simulink library "lib_Clutch_2017a"  (R2017a)
settings: Solver=VariableStepAuto  StartTime=0.0  StopTime=10.0  RelTol=1e-3
settings Model: Creator=leste  LastModifiedBy=Di Russo

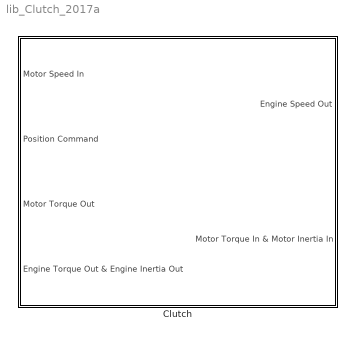
== system lib_Clutch_2017a ==
  Clutch : Subsystem
      mask Display:
      | color('red');
      | port_label('Input',1,'Motor Speed In')
      | port_label('Input',2,'Position Command')
      | port_label('Input',3,'Motor Torque Out')
      | port_label('Input',4,'Engine Trq & Inertia Out')
      | port_label('Output',1,'Engine Speed Out')
      | port_label('Output',2,'Motor Trq Inertia In')

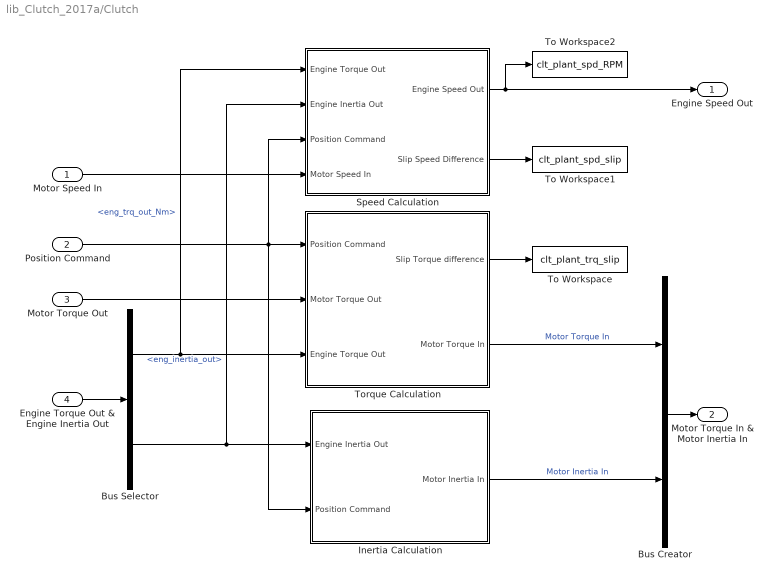
== system lib_Clutch_2017a/Clutch ==
  Motor Speed In : Inport
  Position Command : Inport  Port=2
  Motor Torque Out : Inport  Port=3
  Engine Torque Out & Engine Inertia Out : Inport  Port=4
  Bus Creator : BusCreator  Inputs=2
  Bus Selector : BusSelector  OutputSignals=eng_trq_out_Nm,eng_inertia_out
  Inertia Calculation : Subsystem
  Speed Calculation : Subsystem
  To Workspace : ToWorkspace  VariableName=clt_plant_trq_slip  SaveFormat=Timeseries  SampleTime=-1
  To Workspace1 : ToWorkspace  VariableName=clt_plant_spd_slip  SaveFormat=Timeseries  SampleTime=-1
  To Workspace2 : ToWorkspace  VariableName=clt_plant_spd_RPM  SaveFormat=Timeseries  SampleTime=-1
  Torque Calculation : Subsystem
  Engine Speed Out : Outport
  Motor Torque In & Motor Inertia In : Outport  Port=2
  wires:
  Motor Speed In/1 -> Speed Calculation/4(Motor Speed In)
  Motor Torque Out/1 -> Torque Calculation/2(Motor Torque Out)
  Speed Calculation/2(Slip Speed Difference) -> To Workspace1/1
  Bus Creator/1 -> Motor Torque In & Motor Inertia In/1
  Torque Calculation/1(Slip Torque difference) -> To Workspace/1
  Engine Torque Out & Engine Inertia Out/1 -> Bus Selector/1
  Inertia Calculation/1(Motor Inertia In) -> Bus Creator/2  "Motor Inertia In"
  Torque Calculation/2(Motor Torque In) -> Bus Creator/1  "Motor Torque In"
  Speed Calculation/1(Engine Speed Out) -> Engine Speed Out/1, To Workspace2/1
  Bus Selector/1 -> Torque Calculation/3(Engine Torque Out), Speed Calculation/1(Engine Torque Out)  "<eng_trq_out_Nm>"
  Position Command/1 -> Inertia Calculation/2(Position Command), Speed Calculation/3(Position Command), Torque Calculation/1(Position Command)
  Bus Selector/2 -> Speed Calculation/2(Engine Inertia Out), Inertia Calculation/1(Engine Inertia Out)  "<eng_inertia_out>"

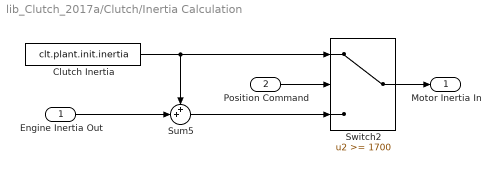
== system lib_Clutch_2017a/Clutch/Inertia Calculation ==
  Engine Inertia Out : Inport
  Position Command : Inport  Port=2
  Clutch Inertia : Constant  Value=clt.plant.init.inertia
  Sum5 : Sum  Inputs=++|  SaturateOnIntegerOverflow=on  InputSameDT=on  OutDataTypeStr=Inherit: Same as first input
  Switch2 : Switch  Threshold=1700  SaturateOnIntegerOverflow=on  InputSameDT=on
  Motor Inertia In : Outport
  wires:
  Clutch Inertia/1 -> Switch2/1, Sum5/1
  Engine Inertia Out/1 -> Sum5/2
  Position Command/1 -> Switch2/2
  Sum5/1 -> Switch2/3
  Switch2/1 -> Motor Inertia In/1

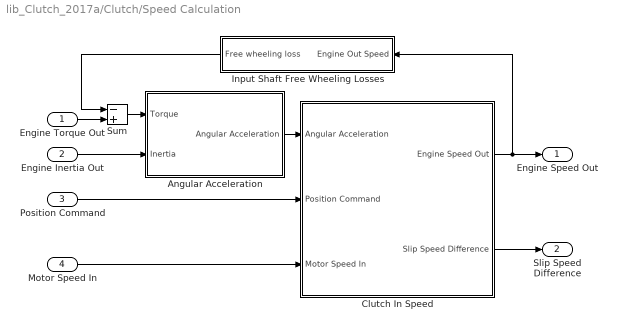
== system lib_Clutch_2017a/Clutch/Speed Calculation ==
  Engine Torque Out : Inport
  Engine Inertia Out : Inport  Port=2
  Position Command : Inport  Port=3
  Motor Speed In : Inport  Port=4
  Angular Acceleration : Subsystem
  "Clutch In Speed " : Subsystem
  Input Shaft Free Wheeling Losses : Subsystem
  Sum : Sum  Inputs=-+
  Engine Speed Out : Outport
  Slip Speed Difference : Outport  Port=2
  wires:
  "Clutch In Speed "/2(Slip Speed Difference) -> Slip Speed Difference/1
  Angular Acceleration/1(Angular Acceleration) -> "Clutch In Speed "/1(Angular Acceleration)
  Position Command/1 -> "Clutch In Speed "/2(Position Command)
  Motor Speed In/1 -> "Clutch In Speed "/3(Motor Speed In)
  Engine Inertia Out/1 -> Angular Acceleration/2(Inertia)
  Engine Torque Out/1 -> Sum/2
  "Clutch In Speed "/1(Engine Speed Out) -> Engine Speed Out/1, Input Shaft Free Wheeling Losses/1(Engine Out Speed)
  Input Shaft Free Wheeling Losses/1(Free wheeling loss) -> Sum/1
  Sum/1 -> Angular Acceleration/1(Torque)

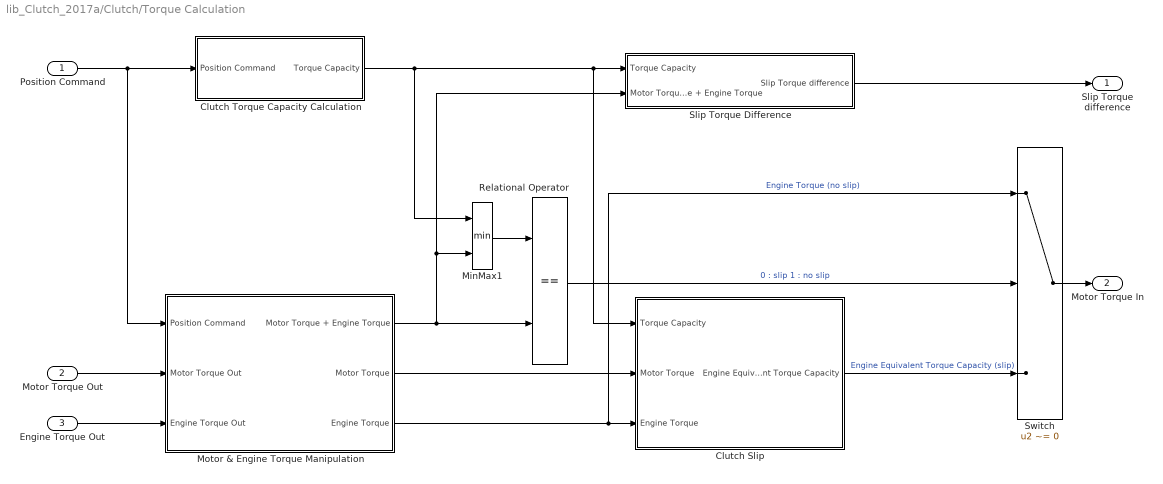
== system lib_Clutch_2017a/Clutch/Torque Calculation ==
  Position Command : Inport
  Motor Torque Out : Inport  Port=2
  Engine Torque Out : Inport  Port=3
  "Clutch Slip " : Subsystem
  Clutch Torque Capacity Calculation : Subsystem
  MinMax1 : MinMax  Inputs=2
  Motor & Engine Torque Manipulation : Subsystem
  Relational Operator : RelationalOperator  Operator===  OutDataTypeStr=boolean  RndMeth=Simplest
  Slip Torque Difference : Subsystem
  Switch : Switch  Criteria=u2 ~= 0
  Slip Torque difference : Outport
  Motor Torque In : Outport  Port=2
  wires:
  Slip Torque Difference/1(Slip Torque difference) -> Slip Torque difference/1
  Motor & Engine Torque Manipulation/2(Motor Torque) -> "Clutch Slip "/2(Motor Torque)
  Engine Torque Out/1 -> Motor & Engine Torque Manipulation/3(Engine Torque Out)
  Motor Torque Out/1 -> Motor & Engine Torque Manipulation/2(Motor Torque Out)
  Motor & Engine Torque Manipulation/3(Engine Torque) -> Switch/1, "Clutch Slip "/3(Engine Torque)  "Engine Torque (no slip)"
  Motor & Engine Torque Manipulation/1(Motor Torque + Engine Torque) -> Slip Torque Difference/2(Motor Torque + Engine Torque), MinMax1/2, Relational Operator/2
  "Clutch Slip "/1(Engine Equivalent Torque Capacity) -> Switch/3  "Engine Equivalent Torque Capacity (slip)"
  Clutch Torque Capacity Calculation/1(Torque Capacity) -> Slip Torque Difference/1(Torque Capacity), "Clutch Slip "/1(Torque Capacity), MinMax1/1
  MinMax1/1 -> Relational Operator/1
  Relational Operator/1 -> Switch/2  "0 : slip 1 : no slip"
  Switch/1 -> Motor Torque In/1
  Position Command/1 -> Motor & Engine Torque Manipulation/1(Position Command), Clutch Torque Capacity Calculation/1(Position Command)

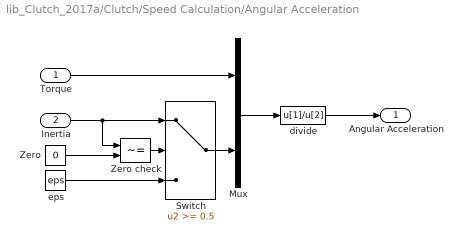
== system lib_Clutch_2017a/Clutch/Speed Calculation/Angular Acceleration ==
  Torque : Inport
  Inertia : Inport  Port=2
  Mux : Mux  Inputs=2
  Switch : Switch  Threshold=0.5  SaturateOnIntegerOverflow=on  InputSameDT=on
  Zero : Constant  Value=0
  Zero check : RelationalOperator  Operator=~=  RndMeth=Nearest  InputSameDT=on
  divide : Fcn  Expr=u[1]/u[2]
  eps : Constant  Value=eps
  Angular Acceleration : Outport
  wires:
  Switch/1 -> Mux/2
  Zero check/1 -> Switch/2
  Zero/1 -> Zero check/2
  eps/1 -> Switch/3
  Inertia/1 -> Zero check/1, Switch/1
  Torque/1 -> Mux/1
  Mux/1 -> divide/1
  divide/1 -> Angular Acceleration/1

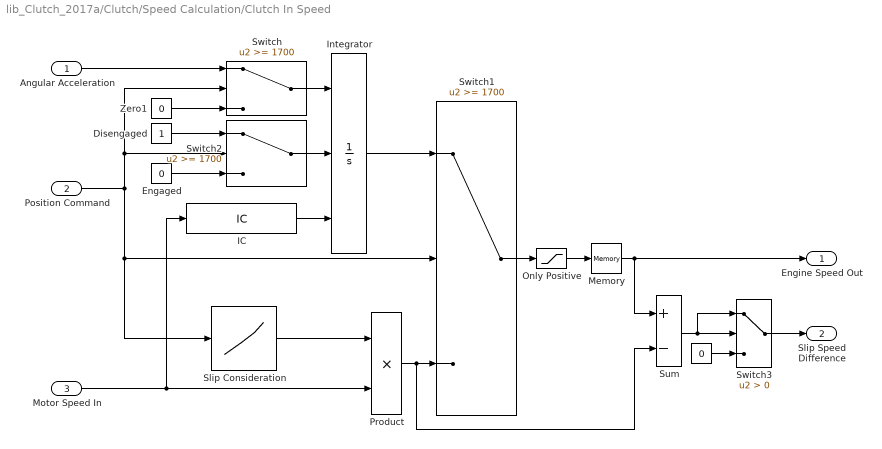
== system lib_Clutch_2017a/Clutch/Speed Calculation/Clutch In Speed  ==
  Angular Acceleration : Inport
  Position Command : Inport  Port=2
  Motor Speed In : Inport  Port=3
  " " : Constant  Value=0
  Disengaged : Constant
  Engaged : Constant  Value=0
  IC : InitialCondition  Value=clt.plant.init.spd_idle
  Integrator : Integrator  ExternalReset=either  InitialConditionSource=external  LimitOutput=on  LowerSaturationLimit=0  AbsoluteTolerance=1e-3
  Memory : Memory
  Only Positive : Saturate  UpperLimit=inf  LowerLimit=0
  Product : Product
  Slip Consideration : Lookup_n-D  NumberOfTableDimensions=1  BreakpointsForDimension1=|  Table=|  InternalRulePriority=Speed  RndMeth=Simplest  InputSameDT=on
      BreakpointsForDimension1=|
      | [0
      | 100
      | 200
      | 300
      | 400
      | 500
      | 600
      | 700
      | 800
      | 900
      | 1000
      | 1100
      | 1200
      | 1300
      | 1400
      | 1500
      | 1600
      | 1700
      | 1800
      | 1900
      | 2000
      | 2100
      | 2200
      | 2300
      | 2400
      | 2500
      | 2600
      | 2700
      | 2800
      | 2900
      | 3000
      | 3100
      | 3200
      | 3300
      | 3400
      | 3500
      | 3600
      | 3700
      | 3800
      | 3900
      | 4000
      | 4100
      | 4200
      | 4300
      | 4400
      | 4500
      | 4600
      | 4700
      | 4800
      | 4900
      | 5000
      | 5100
      | 5200
      | 5300
      | 5400
      | 5500
      | 5600
      | 5700
      | 5800
      | 5900
      | 6000
      | 6100
      | 6200
      | 6300
      | 6400]
      Table=|
      | [1
      | 1
      | 1
      | 0.934
      | 0.868
      | 0.802
      | 0.736
      | 0.67
      | 0.604
      | 0.538
      | 0.472
      | 0.406
      | 0.34
      | 0.274
      | 0.208
      | 0.142
      | 0.076
      | 0
      | 0
      | 0
      | 0
      | 0
      | 0
      | 0
      | 0
      | 0
      | 0
      | 0
      | 0
      | 0
      | 0
      | 0
      | 0
      | 0
      | 0
      | 0
      | 0
      | 0
      | 0
      | 0
      | 0
      | 0
      | 0
      | 0
      | 0
      | 0
      | 0
      | 0
      | 0
      | 0
      | 0
      | 0
      | 0
      | 0
      | 0
      | 0
      | 0
      | 0
      | 0
      | 0
      | 0
      | 0
      | 0
      | 0
      | 0]
  Sum : Sum  Inputs=+-
  Switch : Switch  Threshold=1700  SaturateOnIntegerOverflow=on  InputSameDT=on
  Switch1 : Switch  Threshold=1700  SaturateOnIntegerOverflow=on  InputSameDT=on
  Switch2 : Switch  Threshold=1700  SaturateOnIntegerOverflow=on  InputSameDT=on
  Switch3 : Switch  Criteria=u2 > Threshold  SaturateOnIntegerOverflow=on  InputSameDT=on
  Zero1 : Constant  Value=0
  Engine Speed Out : Outport
  Slip Speed Difference : Outport  Port=2
  wires:
  Only Positive/1 -> Memory/1
  Switch3/1 -> Slip Speed Difference/1
  " "/1 -> Switch3/3
  Sum/1 -> Switch3/2, Switch3/1
  Product/1 -> Switch1/3, Sum/2
  Switch1/1 -> Only Positive/1
  Memory/1 -> Engine Speed Out/1, Sum/1
  Motor Speed In/1 -> IC/1, Product/2
  Switch/1 -> Integrator/1
  Angular Acceleration/1 -> Switch/1
  Integrator/1 -> Switch1/1
  IC/1 -> Integrator/3
  Slip Consideration/1 -> Product/1
  Disengaged/1 -> Switch2/1
  Switch2/1 -> Integrator/2
  Position Command/1 -> Switch/2, Switch2/2, Switch1/2, Slip Consideration/1
  Engaged/1 -> Switch2/3
  Zero1/1 -> Switch/3

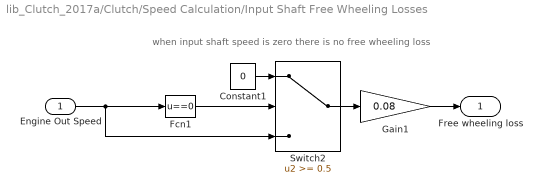
== system lib_Clutch_2017a/Clutch/Speed Calculation/Input Shaft Free Wheeling Losses ==
  note: when input shaft speed is zero there is no free wheeling loss
  Engine Out Speed : Inport
  Constant1 : Constant  Value=0
  Fcn1 : Fcn  Expr=u==0
  Gain1 : Gain  Gain=0.08  SaturateOnIntegerOverflow=on  OutDataTypeStr=Inherit: Same as input  ParamDataTypeStr=Inherit: Same as input
  Switch2 : Switch  Threshold=0.5  SaturateOnIntegerOverflow=on  InputSameDT=on
  Free wheeling loss : Outport
  wires:
  Engine Out Speed/1 -> Switch2/3, Fcn1/1
  Fcn1/1 -> Switch2/2
  Gain1/1 -> Free wheeling loss/1
  Switch2/1 -> Gain1/1
  Constant1/1 -> Switch2/1

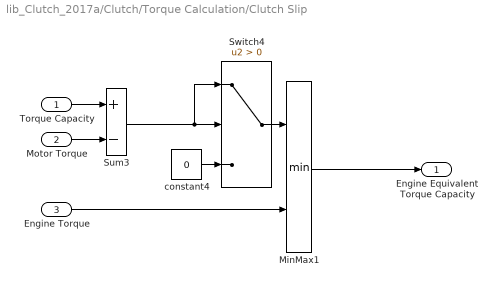
== system lib_Clutch_2017a/Clutch/Torque Calculation/Clutch Slip  ==
  Torque Capacity : Inport
  Motor Torque : Inport  Port=2
  Engine Torque : Inport  Port=3
  MinMax1 : MinMax  Inputs=2
  Sum3 : Sum  Inputs=+-
  Switch4 : Switch  Criteria=u2 > Threshold
  constant4 : Constant  Value=0
  Engine Equivalent Torque Capacity : Outport
  wires:
  Engine Torque/1 -> MinMax1/2
  Motor Torque/1 -> Sum3/2
  Torque Capacity/1 -> Sum3/1
  constant4/1 -> Switch4/3
  Sum3/1 -> Switch4/2, Switch4/1
  Switch4/1 -> MinMax1/1
  MinMax1/1 -> Engine Equivalent Torque Capacity/1

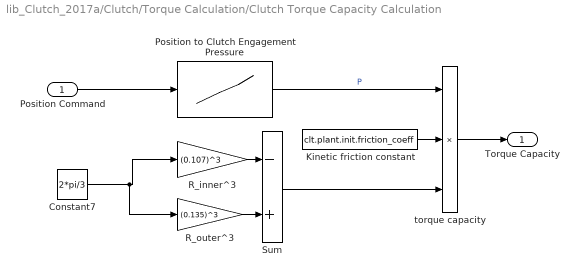
== system lib_Clutch_2017a/Clutch/Torque Calculation/Clutch Torque Capacity Calculation ==
  Position Command : Inport
  Constant7 : Constant  Value=2*pi/3
  Kinetic friction constant : Constant  Value=clt.plant.init.friction_coeff
  Position to Clutch Engagement Pressure : Lookup_n-D  NumberOfTableDimensions=1  BreakpointsForDimension1=|  Table=|  InternalRulePriority=Speed  RndMeth=Simplest  InputSameDT=on
      BreakpointsForDimension1=|
      | [0
      | 100
      | 200
      | 300
      | 400
      | 500
      | 600
      | 700
      | 800
      | 900
      | 1000
      | 1100
      | 1200
      | 1300
      | 1400
      | 1500
      | 1600
      | 1700
      | 1800
      | 1900
      | 2000
      | 2100
      | 2200
      | 2300
      | 2400
      | 2500
      | 2600
      | 2700
      | 2800
      | 2900
      | 3000
      | 3100
      | 3200
      | 3300
      | 3400
      | 3500
      | 3600
      | 3700
      | 3800
      | 3900
      | 4000
      | 4100
      | 4200
      | 4300
      | 4400
      | 4500
      | 4600
      | 4700
      | 4800
      | 4900
      | 5000
      | 5100
      | 5200
      | 5300
      | 5400
      | 5500
      | 5600
      | 5700
      | 5800
      | 5900
      | 6000
      | 6100
      | 6200
      | 6300
      | 6400
      | 
      | ]
      Table=|
      | [892800
      | 892800
      | 892800
      | 833280
      | 773760
      | 714240
      | 654720
      | 595200
      | 535680
      | 476160
      | 416640
      | 357120
      | 297600
      | 238080
      | 178560
      | 119040
      | 59520
      | 0
      | 0
      | 0
      | 0
      | 0
      | 0
      | 0
      | 0
      | 0
      | 0
      | 0
      | 0
      | 0
      | 0
      | 0
      | 0
      | 0
      | 0
      | 0
      | 0
      | 0
      | 0
      | 0
      | 0
      | 0
      | 0
      | 0
      | 0
      | 0
      | 0
      | 0
      | 0
      | 0
      | 0
      | 0
      | 0
      | 0
      | 0
      | 0
      | 0
      | 0
      | 0
      | 0
      | 0
      | 0
      | 0
      | 0
      | 0
      | 
      | 
      | ]
  R_inner^3 : Gain  Gain=(0.107)^3
  R_outer^3 : Gain  Gain=(0.135)^3
  Sum : Sum  Inputs=-+
  torque capacity : Product  Inputs=3  SaturateOnIntegerOverflow=on  InputSameDT=on  OutDataTypeStr=Inherit: Same as first input
  Torque Capacity : Outport
  wires:
  Constant7/1 -> R_inner^3/1, R_outer^3/1
  Position Command/1 -> Position to Clutch Engagement Pressure/1
  torque capacity/1 -> Torque Capacity/1
  Position to Clutch Engagement Pressure/1 -> torque capacity/1  "P"
  R_outer^3/1 -> Sum/2
  Sum/1 -> torque capacity/3
  Kinetic friction constant/1 -> torque capacity/2
  R_inner^3/1 -> Sum/1

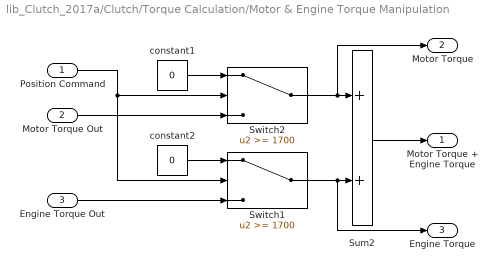
== system lib_Clutch_2017a/Clutch/Torque Calculation/Motor & Engine Torque Manipulation ==
  Position Command : Inport
  Motor Torque Out : Inport  Port=2
  Engine Torque Out : Inport  Port=3
  Sum2 : Sum
  Switch1 : Switch  Threshold=1700
  Switch2 : Switch  Threshold=1700
  constant1 : Constant  Value=0
  constant2 : Constant  Value=0
  Motor Torque + Engine Torque : Outport
  Motor Torque : Outport  Port=2
  Engine Torque : Outport  Port=3
  wires:
  Position Command/1 -> Switch2/2, Switch1/2
  Switch2/1 -> Sum2/1, Motor Torque/1
  Sum2/1 -> Motor Torque + Engine Torque/1
  constant2/1 -> Switch1/1
  Switch1/1 -> Sum2/2, Engine Torque/1
  constant1/1 -> Switch2/1
  Engine Torque Out/1 -> Switch1/3
  Motor Torque Out/1 -> Switch2/3

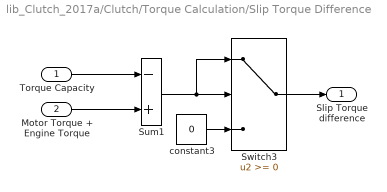
== system lib_Clutch_2017a/Clutch/Torque Calculation/Slip Torque Difference ==
  Torque Capacity : Inport
  Motor Torque + Engine Torque : Inport  Port=2
  Sum1 : Sum  Inputs=-+
  Switch3 : Switch
  constant3 : Constant  Value=0
  Slip Torque difference : Outport
  wires:
  Torque Capacity/1 -> Sum1/1
  Motor Torque + Engine Torque/1 -> Sum1/2
  Switch3/1 -> Slip Torque difference/1
  constant3/1 -> Switch3/3
  Sum1/1 -> Switch3/2, Switch3/1
